simulink model "regulator_de_stare"  (R2023b)
settings: Solver=VariableStepAuto  StartTime=0.0  StopTime=200  RelTol=1e-3
settings Model: Creator=Iustin  LastModifiedBy=Iustin

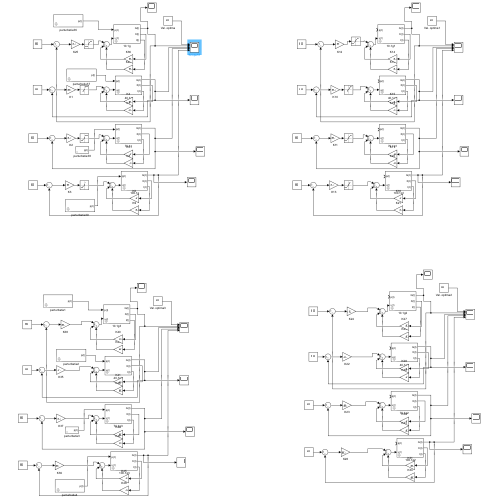
[thumbnail: Simulink's stored preview of the top-level diagram]
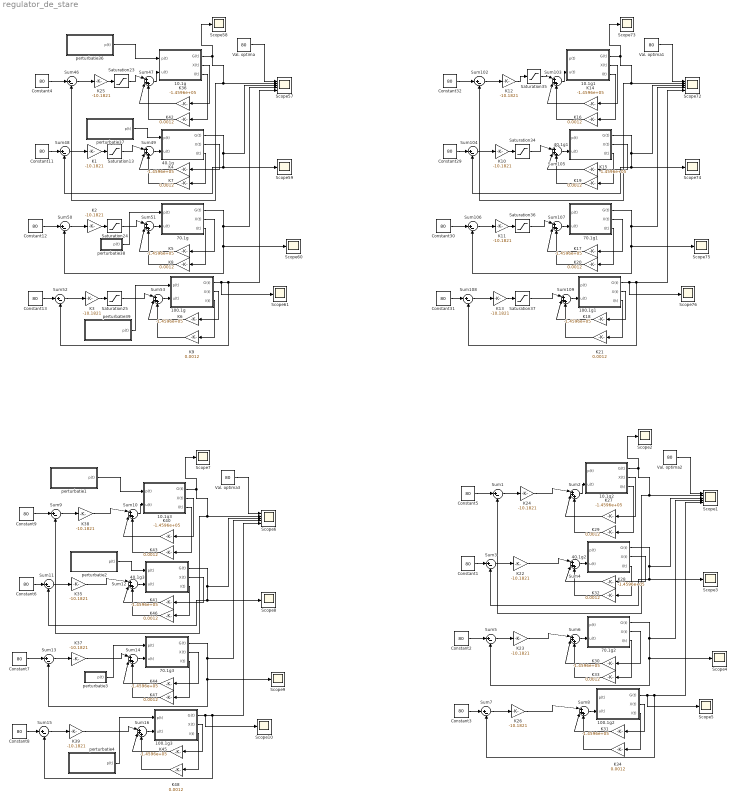
== system regulator_de_stare ==
  " 100.1g" : Subsystem  mask{Gb=80, V=120, p1=0.032, p2=0.019, p3=0.00000987, n=0.208, G0=100}
  " 100.1g1" : Subsystem  mask{Gb=80, V=120, p1=0.032, p2=0.019, p3=0.00000987, n=0.208, G0=300}
  " 100.1g2" : Subsystem  mask{Gb=80, V=120, p1=0.032, p2=0.019, p3=0.00000987, n=0.208, G0=300}
  " 100.1g3" : Subsystem  mask{Gb=80, V=120, p1=0.032, p2=0.019, p3=0.00000987, n=0.208, G0=100}
  10.1g : Subsystem  mask{Gb=80, V=120, p1=0.032, p2=0.019, p3=0.00000987, n=0.208, G0=100}
  10.1g1 : Subsystem  mask{Gb=80, V=120, p1=0.032, p2=0.019, p3=0.00000987, n=0.208, G0=150}
  10.1g2 : Subsystem  mask{Gb=80, V=120, p1=0.032, p2=0.019, p3=0.00000987, n=0.208, G0=150}
  10.1g3 : Subsystem  mask{Gb=80, V=120, p1=0.032, p2=0.019, p3=0.00000987, n=0.208, G0=100}
  40.1g : Subsystem  mask{Gb=80, V=120, p1=0.032, p2=0.019, p3=0.00000987, n=0.208, G0=100}
  40.1g1 : Subsystem  mask{Gb=80, V=120, p1=0.032, p2=0.019, p3=0.00000987, n=0.208, G0=200}
  40.1g2 : Subsystem  mask{Gb=80, V=120, p1=0.032, p2=0.019, p3=0.00000987, n=0.208, G0=200}
  40.1g3 : Subsystem  mask{Gb=80, V=120, p1=0.032, p2=0.019, p3=0.00000987, n=0.208, G0=100}
  70.1g : Subsystem  mask{Gb=80, V=120, p1=0.032, p2=0.019, p3=0.00000987, n=0.208, G0=100}
  70.1g1 : Subsystem  mask{Gb=80, V=120, p1=0.032, p2=0.019, p3=0.00000987, n=0.208, G0=250}
  70.1g2 : Subsystem  mask{Gb=80, V=120, p1=0.032, p2=0.019, p3=0.00000987, n=0.208, G0=250}
  70.1g3 : Subsystem  mask{Gb=80, V=120, p1=0.032, p2=0.019, p3=0.00000987, n=0.208, G0=100}
  Constant{1..9,11..13,29..32} (16 alike) : Constant  Value=80
  K{1..3,10..13,22..26,35,37..39} (16 alike) : Gain  Gain=-10.1821
  K{4..6,14..15,17..18,27..28,30..31,36,40..41,44..45} (16 alike) : Gain  Gain=-1.4596e+05
  K{7..9,16,19..21,29,32..34,42..43,46..48} (16 alike) : Gain  Gain=0.0012
  Saturation{13,23..25,34..37} (8 alike) : Saturate  UpperLimit=500  LowerLimit=0
  Scope{1,6,57,72} (4 alike) : Scope  NumInputPorts=5
  Scope{2..5,7..10,58..61,73..76} (16 alike) : Scope
  Sum{1,3,5,7,9,11,13,15,46,48,50,52,102,104,106,108} (16 alike) : Sum  Inputs=|+-
  Sum{2,4,6,8,10,12,14,16,47,49,51,53,103,105,107,109} (16 alike) : Sum  Inputs=|+++
  Val. optima{,1..3} (4 alike) : Constant  Value=80
  perturbatie1 : Subsystem  mask{Dg=10*1000, Ag=0.8, tg_max=40}
  perturbatie2 : Subsystem  mask{Dg=40*1000, Ag=0.8, tg_max=40}
  perturbatie3 : Subsystem  mask{Dg=70*1000, Ag=0.8, tg_max=40}
  perturbatie36 : Subsystem  mask{Dg=10*1000, Ag=0.8, tg_max=40}
  perturbatie37 : Subsystem  mask{Dg=40*1000, Ag=0.8, tg_max=40}
  perturbatie38 : Subsystem  mask{Dg=70*1000, Ag=0.8, tg_max=40}
  perturbatie39 : Subsystem  mask{Dg=100*1000, Ag=0.8, tg_max=40}
  perturbatie4 : Subsystem  mask{Dg=100*1000, Ag=0.8, tg_max=40}
  wires:
  70.1g1/2(X(t)) -> K17/1
  K16/1 -> Sum103/3
  40.1g1/2(X(t)) -> K15/1
  Sum107/1 -> 70.1g1/2(u(t))
  K19/1 -> Sum105/3
  K14/1 -> Sum103/2
  40.1g1/1(G(t)) -> Scope72/3, Scope74/1, Sum104/2
  Constant30/1 -> Sum106/1
  10.1g1/2(X(t)) -> K14/1
  Saturation34/1 -> Sum105/1
  " 100.1g1"/3(I(t)) -> K21/1
  70.1g1/1(G(t)) -> Scope72/4, Scope75/1, Sum106/2
  " 100.1g1"/2(X(t)) -> K18/1
  40.1g1/3(I(t)) -> K19/1
  Constant32/1 -> Sum102/1
  Sum103/1 -> 10.1g1/2(u(t))
  70.1g1/3(I(t)) -> K20/1
  " 100.1g1"/1(G(t)) -> Scope76/1, Scope72/5, Sum108/2
  Sum109/1 -> " 100.1g1"/2(u(t))
  Sum105/1 -> 40.1g1/2(u(t))
  Sum104/1 -> K10/1
  Constant31/1 -> Sum108/1
  K18/1 -> Sum109/2
  K10/1 -> Saturation34/1
  Sum106/1 -> K11/1
  10.1g1/1(G(t)) -> Sum102/2, Scope72/2, Scope73/1
  K11/1 -> Saturation36/1
  Val. optima1/1 -> Scope72/1
  Saturation37/1 -> Sum109/1
  K20/1 -> Sum107/3
  K8/1 -> Sum51/3
  K21/1 -> Sum109/3
  Sum108/1 -> K13/1
  Saturation36/1 -> Sum107/1
  K17/1 -> Sum107/2
  40.1g/3(I(t)) -> K7/1
  Sum51/1 -> 70.1g/2(u(t))
  10.1g/2(X(t)) -> K36/1
  70.1g/1(G(t)) -> Scope57/4, Scope60/1, Sum50/2
  Val. optima/1 -> Scope57/1
  Sum46/1 -> K25/1
  Saturation23/1 -> Sum47/1
  Saturation13/1 -> Sum49/1
  70.1g/3(I(t)) -> K8/1
  Constant4/1 -> Sum46/1
  Constant11/1 -> Sum48/1
  K4/1 -> Sum49/2
  70.1g/2(X(t)) -> K5/1
  K5/1 -> Sum51/2
  K15/1 -> Sum105/2
  Saturation25/1 -> Sum53/1
  K36/1 -> Sum47/2
  K3/1 -> Saturation25/1
  40.1g/1(G(t)) -> Scope57/3, Scope59/1, Sum48/2
  perturbatie39/1(p(t)) -> " 100.1g"/1(p(t))
  K6/1 -> Sum53/2
  Saturation24/1 -> Sum51/1
  K7/1 -> Sum49/3
  K25/1 -> Saturation23/1
  perturbatie38/1(p(t)) -> 70.1g/1(p(t))
  Sum102/1 -> K12/1
  perturbatie36/1(p(t)) -> 10.1g/1(p(t))
  K42/1 -> Sum47/3
  Constant12/1 -> Sum50/1
  10.1g/3(I(t)) -> K42/1
  Constant29/1 -> Sum104/1
  " 100.1g"/3(I(t)) -> K9/1
  Sum47/1 -> 10.1g/2(u(t))
  K9/1 -> Sum53/3
  K1/1 -> Saturation13/1
  Sum53/1 -> " 100.1g"/2(u(t))
  K2/1 -> Saturation24/1
  K13/1 -> Saturation37/1
  Sum49/1 -> 40.1g/2(u(t))
  Constant13/1 -> Sum52/1
  perturbatie37/1(p(t)) -> 40.1g/1(p(t))
  Sum52/1 -> K3/1
  40.1g/2(X(t)) -> K4/1
  " 100.1g"/2(X(t)) -> K6/1
  Sum48/1 -> K1/1
  Sum50/1 -> K2/1
  K12/1 -> Saturation35/1
  10.1g1/3(I(t)) -> K16/1
  10.1g/1(G(t)) -> Sum46/2, Scope57/2, Scope58/1
  Saturation35/1 -> Sum103/1
  " 100.1g"/1(G(t)) -> Scope61/1, Scope57/5, Sum52/2
  Sum4/1 -> 40.1g2/2(u(t))
  K23/1 -> Sum6/1
  K26/1 -> Sum8/1
  70.1g2/1(G(t)) -> Scope1/4, Scope4/1, Sum5/2
  Sum8/1 -> " 100.1g2"/2(u(t))
  " 100.1g2"/1(G(t)) -> Scope5/1, Scope1/5, Sum7/2
  70.1g2/3(I(t)) -> K33/1
  40.1g2/3(I(t)) -> K32/1
  Sum3/1 -> K22/1
  " 100.1g2"/3(I(t)) -> K34/1
  10.1g2/1(G(t)) -> Sum1/2, Scope1/2, Scope2/1
  Constant1/1 -> Sum3/1
  " 100.1g2"/2(X(t)) -> K31/1
  Sum5/1 -> K23/1
  Sum6/1 -> 70.1g2/2(u(t))
  K31/1 -> Sum8/2
  10.1g2/2(X(t)) -> K27/1
  40.1g2/1(G(t)) -> Scope1/3, Scope3/1, Sum3/2
  K28/1 -> Sum4/2
  K29/1 -> Sum2/3
  K22/1 -> Sum4/1
  K32/1 -> Sum4/3
  70.1g2/2(X(t)) -> K30/1
  40.1g2/2(X(t)) -> K28/1
  Constant5/1 -> Sum1/1
  Constant2/1 -> Sum5/1
  K27/1 -> Sum2/2
  K30/1 -> Sum6/2
  10.1g2/3(I(t)) -> K29/1
  Val. optima2/1 -> Scope1/1
  K33/1 -> Sum6/3
  K24/1 -> Sum2/1
  Sum1/1 -> K24/1
  Sum2/1 -> 10.1g2/2(u(t))
  Sum7/1 -> K26/1
  K34/1 -> Sum8/3
  Constant3/1 -> Sum7/1
  70.1g3/1(G(t)) -> Scope6/4, Scope9/1, Sum13/2
  Sum10/1 -> 10.1g3/2(u(t))
  " 100.1g3"/3(I(t)) -> K48/1
  Val. optima3/1 -> Scope6/1
  K35/1 -> Sum12/1
  40.1g3/3(I(t)) -> K46/1
  K38/1 -> Sum10/1
  Constant6/1 -> Sum11/1
  K39/1 -> Sum16/1
  K40/1 -> Sum10/2
  Sum13/1 -> K37/1
  K41/1 -> Sum12/2
  Sum11/1 -> K35/1
  Sum12/1 -> 40.1g3/2(u(t))
  Sum15/1 -> K39/1
  Sum16/1 -> " 100.1g3"/2(u(t))
  K46/1 -> Sum12/3
  40.1g3/1(G(t)) -> Scope6/3, Scope8/1, Sum11/2
  40.1g3/2(X(t)) -> K41/1
  Constant8/1 -> Sum15/1
  Sum9/1 -> K38/1
  perturbatie3/1(p(t)) -> 70.1g3/1(p(t))
  K44/1 -> Sum14/2
  70.1g3/3(I(t)) -> K47/1
  Constant7/1 -> Sum13/1
  K37/1 -> Sum14/1
  K43/1 -> Sum10/3
  perturbatie4/1(p(t)) -> " 100.1g3"/1(p(t))
  10.1g3/2(X(t)) -> K40/1
  K47/1 -> Sum14/3
  Constant9/1 -> Sum9/1
  " 100.1g3"/2(X(t)) -> K45/1
  10.1g3/1(G(t)) -> Sum9/2, Scope6/2, Scope7/1
  K45/1 -> Sum16/2
  perturbatie2/1(p(t)) -> 40.1g3/1(p(t))
  Sum14/1 -> 70.1g3/2(u(t))
  10.1g3/3(I(t)) -> K43/1
  perturbatie1/1(p(t)) -> 10.1g3/1(p(t))
  " 100.1g3"/1(G(t)) -> Scope10/1, Scope6/5, Sum15/2
  70.1g3/2(X(t)) -> K44/1
  K48/1 -> Sum16/3

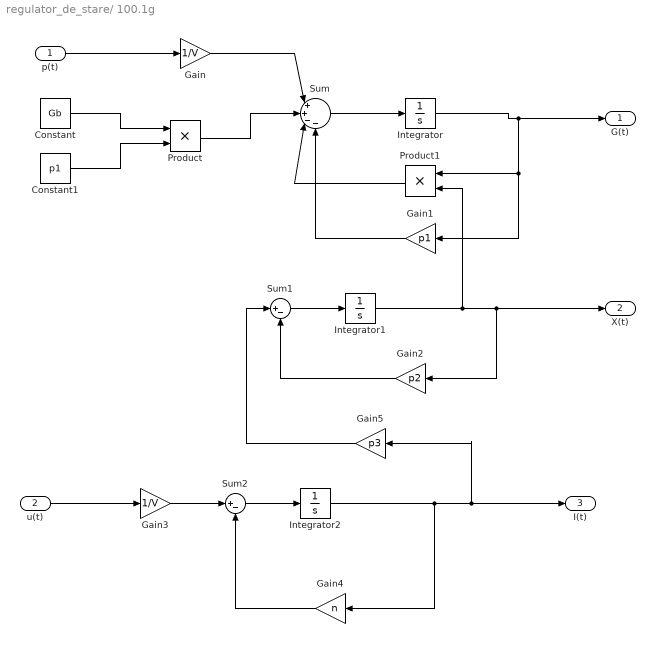
== system regulator_de_stare/ 100.1g ==
  p(t) : Inport
  u(t) : Inport  Port=2
  Constant : Constant  Value=Gb
  Constant1 : Constant  Value=p1
  Gain : Gain  Gain=1/V
  Gain1 : Gain  Gain=p1
  Gain2 : Gain  Gain=p2
  Gain3 : Gain  Gain=1/V
  Gain4 : Gain  Gain=n
  Gain5 : Gain  Gain=p3
  Integrator : Integrator  InitialCondition=G0
  Integrator1 : Integrator
  Integrator2 : Integrator
  Product : Product
  Product1 : Product
  Sum : Sum  Inputs=|++--
  Sum1 : Sum  Inputs=|+-
  Sum2 : Sum  Inputs=|+-
  G(t) : Outport
  X(t) : Outport  Port=2
  I(t) : Outport  Port=3
  wires:
  Sum2/1 -> Integrator2/1
  Gain3/1 -> Sum2/1
  Sum1/1 -> Integrator1/1
  Integrator2/1 -> Gain4/1, I(t)/1, Gain5/1
  u(t)/1 -> Gain3/1
  Integrator1/1 -> Product1/2, X(t)/1, Gain2/1
  Product/1 -> Sum/2
  Integrator/1 -> G(t)/1, Gain1/1, Product1/1
  Gain5/1 -> Sum1/1
  Sum/1 -> Integrator/1
  Constant1/1 -> Product/2
  Constant/1 -> Product/1
  Gain4/1 -> Sum2/2
  Gain2/1 -> Sum1/2
  Product1/1 -> Sum/3
  Gain1/1 -> Sum/4
  p(t)/1 -> Gain/1
  Gain/1 -> Sum/1

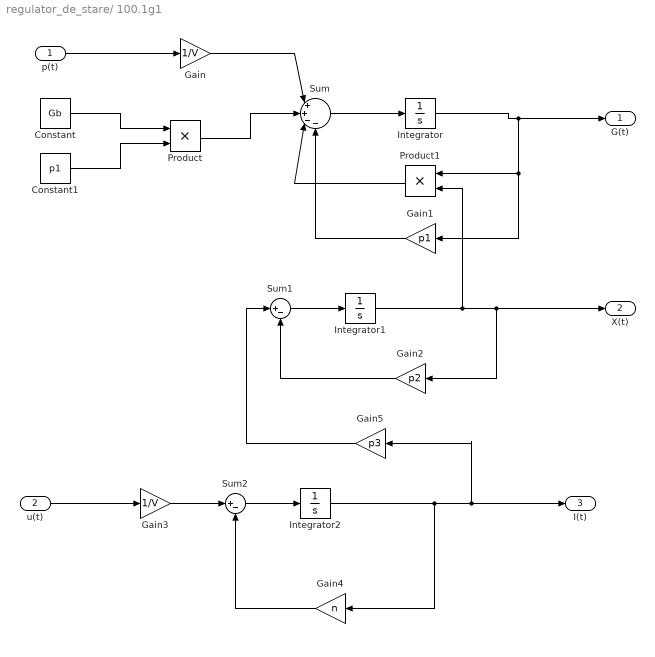
== system regulator_de_stare/ 100.1g1 ==
  p(t) : Inport
  u(t) : Inport  Port=2
  Constant : Constant  Value=Gb
  Constant1 : Constant  Value=p1
  Gain : Gain  Gain=1/V
  Gain1 : Gain  Gain=p1
  Gain2 : Gain  Gain=p2
  Gain3 : Gain  Gain=1/V
  Gain4 : Gain  Gain=n
  Gain5 : Gain  Gain=p3
  Integrator : Integrator  InitialCondition=G0
  Integrator1 : Integrator
  Integrator2 : Integrator
  Product : Product
  Product1 : Product
  Sum : Sum  Inputs=|++--
  Sum1 : Sum  Inputs=|+-
  Sum2 : Sum  Inputs=|+-
  G(t) : Outport
  X(t) : Outport  Port=2
  I(t) : Outport  Port=3
  wires:
  Sum2/1 -> Integrator2/1
  Gain3/1 -> Sum2/1
  Sum1/1 -> Integrator1/1
  Integrator2/1 -> Gain4/1, I(t)/1, Gain5/1
  u(t)/1 -> Gain3/1
  Integrator1/1 -> Product1/2, X(t)/1, Gain2/1
  Product/1 -> Sum/2
  Integrator/1 -> G(t)/1, Gain1/1, Product1/1
  Gain5/1 -> Sum1/1
  Sum/1 -> Integrator/1
  Constant1/1 -> Product/2
  Constant/1 -> Product/1
  Gain4/1 -> Sum2/2
  Gain2/1 -> Sum1/2
  Product1/1 -> Sum/3
  Gain1/1 -> Sum/4
  p(t)/1 -> Gain/1
  Gain/1 -> Sum/1

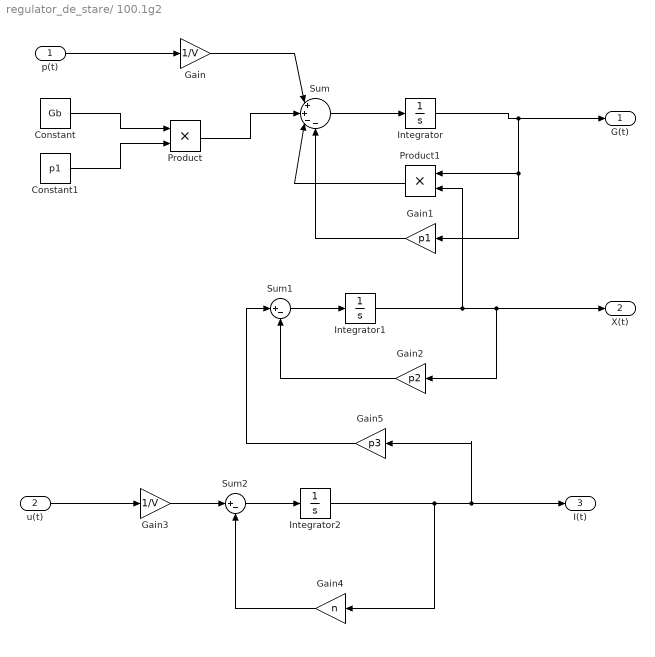
== system regulator_de_stare/ 100.1g2 ==
  p(t) : Inport
  u(t) : Inport  Port=2
  Constant : Constant  Value=Gb
  Constant1 : Constant  Value=p1
  Gain : Gain  Gain=1/V
  Gain1 : Gain  Gain=p1
  Gain2 : Gain  Gain=p2
  Gain3 : Gain  Gain=1/V
  Gain4 : Gain  Gain=n
  Gain5 : Gain  Gain=p3
  Integrator : Integrator  InitialCondition=G0
  Integrator1 : Integrator
  Integrator2 : Integrator
  Product : Product
  Product1 : Product
  Sum : Sum  Inputs=|++--
  Sum1 : Sum  Inputs=|+-
  Sum2 : Sum  Inputs=|+-
  G(t) : Outport
  X(t) : Outport  Port=2
  I(t) : Outport  Port=3
  wires:
  Sum2/1 -> Integrator2/1
  Gain3/1 -> Sum2/1
  Sum1/1 -> Integrator1/1
  Integrator2/1 -> Gain4/1, I(t)/1, Gain5/1
  u(t)/1 -> Gain3/1
  Integrator1/1 -> Product1/2, X(t)/1, Gain2/1
  Product/1 -> Sum/2
  Integrator/1 -> G(t)/1, Gain1/1, Product1/1
  Gain5/1 -> Sum1/1
  Sum/1 -> Integrator/1
  Constant1/1 -> Product/2
  Constant/1 -> Product/1
  Gain4/1 -> Sum2/2
  Gain2/1 -> Sum1/2
  Product1/1 -> Sum/3
  Gain1/1 -> Sum/4
  p(t)/1 -> Gain/1
  Gain/1 -> Sum/1

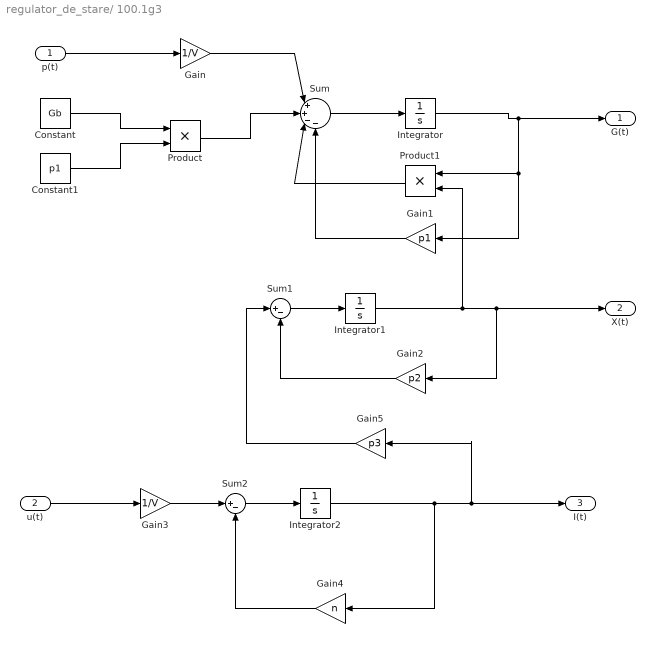
== system regulator_de_stare/ 100.1g3 ==
  p(t) : Inport
  u(t) : Inport  Port=2
  Constant : Constant  Value=Gb
  Constant1 : Constant  Value=p1
  Gain : Gain  Gain=1/V
  Gain1 : Gain  Gain=p1
  Gain2 : Gain  Gain=p2
  Gain3 : Gain  Gain=1/V
  Gain4 : Gain  Gain=n
  Gain5 : Gain  Gain=p3
  Integrator : Integrator  InitialCondition=G0
  Integrator1 : Integrator
  Integrator2 : Integrator
  Product : Product
  Product1 : Product
  Sum : Sum  Inputs=|++--
  Sum1 : Sum  Inputs=|+-
  Sum2 : Sum  Inputs=|+-
  G(t) : Outport
  X(t) : Outport  Port=2
  I(t) : Outport  Port=3
  wires:
  Sum2/1 -> Integrator2/1
  Gain3/1 -> Sum2/1
  Sum1/1 -> Integrator1/1
  Integrator2/1 -> Gain4/1, I(t)/1, Gain5/1
  u(t)/1 -> Gain3/1
  Integrator1/1 -> Product1/2, X(t)/1, Gain2/1
  Product/1 -> Sum/2
  Integrator/1 -> G(t)/1, Gain1/1, Product1/1
  Gain5/1 -> Sum1/1
  Sum/1 -> Integrator/1
  Constant1/1 -> Product/2
  Constant/1 -> Product/1
  Gain4/1 -> Sum2/2
  Gain2/1 -> Sum1/2
  Product1/1 -> Sum/3
  Gain1/1 -> Sum/4
  p(t)/1 -> Gain/1
  Gain/1 -> Sum/1

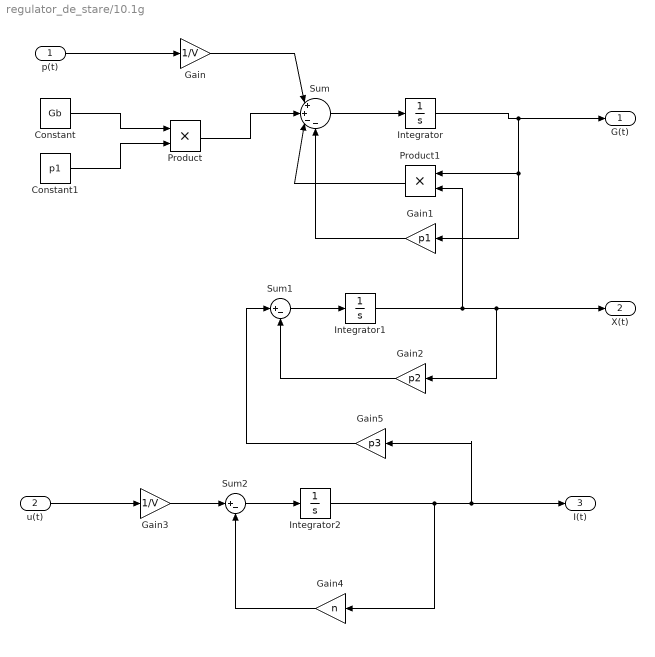
== system regulator_de_stare/10.1g ==
  p(t) : Inport
  u(t) : Inport  Port=2
  Constant : Constant  Value=Gb
  Constant1 : Constant  Value=p1
  Gain : Gain  Gain=1/V
  Gain1 : Gain  Gain=p1
  Gain2 : Gain  Gain=p2
  Gain3 : Gain  Gain=1/V
  Gain4 : Gain  Gain=n
  Gain5 : Gain  Gain=p3
  Integrator : Integrator  InitialCondition=G0
  Integrator1 : Integrator
  Integrator2 : Integrator
  Product : Product
  Product1 : Product
  Sum : Sum  Inputs=|++--
  Sum1 : Sum  Inputs=|+-
  Sum2 : Sum  Inputs=|+-
  G(t) : Outport
  X(t) : Outport  Port=2
  I(t) : Outport  Port=3
  wires:
  Sum2/1 -> Integrator2/1
  Gain3/1 -> Sum2/1
  Sum1/1 -> Integrator1/1
  Integrator2/1 -> Gain4/1, I(t)/1, Gain5/1
  u(t)/1 -> Gain3/1
  Integrator1/1 -> Product1/2, X(t)/1, Gain2/1
  Product/1 -> Sum/2
  Integrator/1 -> G(t)/1, Gain1/1, Product1/1
  Gain5/1 -> Sum1/1
  Sum/1 -> Integrator/1
  Constant1/1 -> Product/2
  Constant/1 -> Product/1
  Gain4/1 -> Sum2/2
  Gain2/1 -> Sum1/2
  Product1/1 -> Sum/3
  Gain1/1 -> Sum/4
  p(t)/1 -> Gain/1
  Gain/1 -> Sum/1

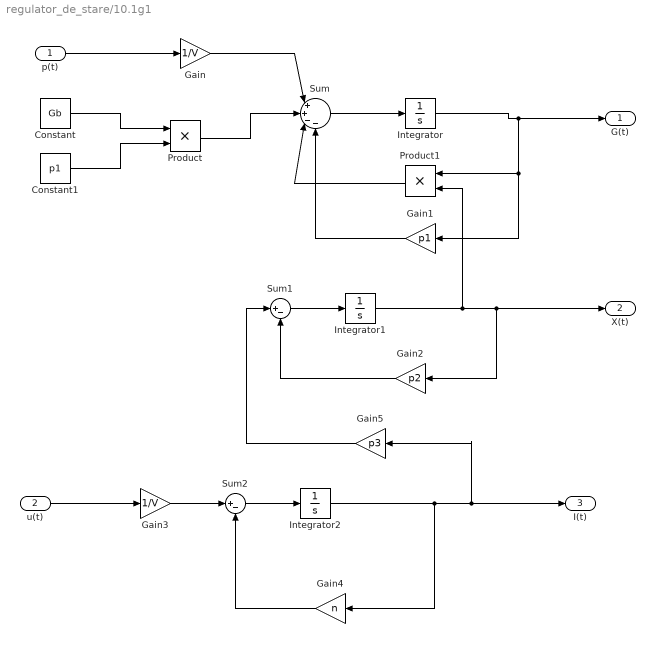
== system regulator_de_stare/10.1g1 ==
  p(t) : Inport
  u(t) : Inport  Port=2
  Constant : Constant  Value=Gb
  Constant1 : Constant  Value=p1
  Gain : Gain  Gain=1/V
  Gain1 : Gain  Gain=p1
  Gain2 : Gain  Gain=p2
  Gain3 : Gain  Gain=1/V
  Gain4 : Gain  Gain=n
  Gain5 : Gain  Gain=p3
  Integrator : Integrator  InitialCondition=G0
  Integrator1 : Integrator
  Integrator2 : Integrator
  Product : Product
  Product1 : Product
  Sum : Sum  Inputs=|++--
  Sum1 : Sum  Inputs=|+-
  Sum2 : Sum  Inputs=|+-
  G(t) : Outport
  X(t) : Outport  Port=2
  I(t) : Outport  Port=3
  wires:
  Sum2/1 -> Integrator2/1
  Gain3/1 -> Sum2/1
  Sum1/1 -> Integrator1/1
  Integrator2/1 -> Gain4/1, I(t)/1, Gain5/1
  u(t)/1 -> Gain3/1
  Integrator1/1 -> Product1/2, X(t)/1, Gain2/1
  Product/1 -> Sum/2
  Integrator/1 -> G(t)/1, Gain1/1, Product1/1
  Gain5/1 -> Sum1/1
  Sum/1 -> Integrator/1
  Constant1/1 -> Product/2
  Constant/1 -> Product/1
  Gain4/1 -> Sum2/2
  Gain2/1 -> Sum1/2
  Product1/1 -> Sum/3
  Gain1/1 -> Sum/4
  p(t)/1 -> Gain/1
  Gain/1 -> Sum/1

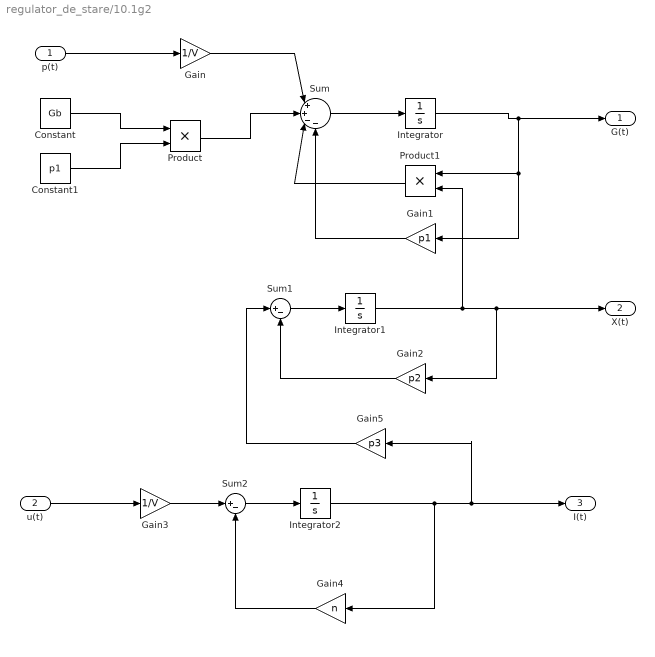
== system regulator_de_stare/10.1g2 ==
  p(t) : Inport
  u(t) : Inport  Port=2
  Constant : Constant  Value=Gb
  Constant1 : Constant  Value=p1
  Gain : Gain  Gain=1/V
  Gain1 : Gain  Gain=p1
  Gain2 : Gain  Gain=p2
  Gain3 : Gain  Gain=1/V
  Gain4 : Gain  Gain=n
  Gain5 : Gain  Gain=p3
  Integrator : Integrator  InitialCondition=G0
  Integrator1 : Integrator
  Integrator2 : Integrator
  Product : Product
  Product1 : Product
  Sum : Sum  Inputs=|++--
  Sum1 : Sum  Inputs=|+-
  Sum2 : Sum  Inputs=|+-
  G(t) : Outport
  X(t) : Outport  Port=2
  I(t) : Outport  Port=3
  wires:
  Sum2/1 -> Integrator2/1
  Gain3/1 -> Sum2/1
  Sum1/1 -> Integrator1/1
  Integrator2/1 -> Gain4/1, I(t)/1, Gain5/1
  u(t)/1 -> Gain3/1
  Integrator1/1 -> Product1/2, X(t)/1, Gain2/1
  Product/1 -> Sum/2
  Integrator/1 -> G(t)/1, Gain1/1, Product1/1
  Gain5/1 -> Sum1/1
  Sum/1 -> Integrator/1
  Constant1/1 -> Product/2
  Constant/1 -> Product/1
  Gain4/1 -> Sum2/2
  Gain2/1 -> Sum1/2
  Product1/1 -> Sum/3
  Gain1/1 -> Sum/4
  p(t)/1 -> Gain/1
  Gain/1 -> Sum/1

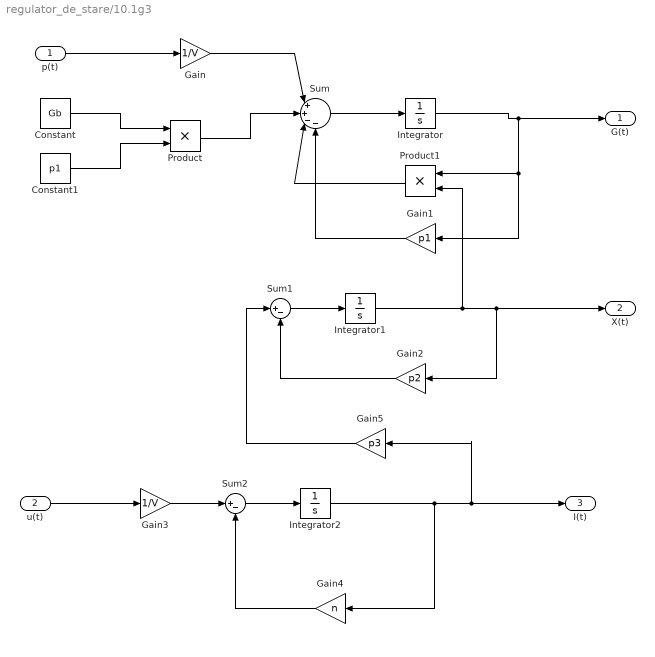
== system regulator_de_stare/10.1g3 ==
  p(t) : Inport
  u(t) : Inport  Port=2
  Constant : Constant  Value=Gb
  Constant1 : Constant  Value=p1
  Gain : Gain  Gain=1/V
  Gain1 : Gain  Gain=p1
  Gain2 : Gain  Gain=p2
  Gain3 : Gain  Gain=1/V
  Gain4 : Gain  Gain=n
  Gain5 : Gain  Gain=p3
  Integrator : Integrator  InitialCondition=G0
  Integrator1 : Integrator
  Integrator2 : Integrator
  Product : Product
  Product1 : Product
  Sum : Sum  Inputs=|++--
  Sum1 : Sum  Inputs=|+-
  Sum2 : Sum  Inputs=|+-
  G(t) : Outport
  X(t) : Outport  Port=2
  I(t) : Outport  Port=3
  wires:
  Sum2/1 -> Integrator2/1
  Gain3/1 -> Sum2/1
  Sum1/1 -> Integrator1/1
  Integrator2/1 -> Gain4/1, I(t)/1, Gain5/1
  u(t)/1 -> Gain3/1
  Integrator1/1 -> Product1/2, X(t)/1, Gain2/1
  Product/1 -> Sum/2
  Integrator/1 -> G(t)/1, Gain1/1, Product1/1
  Gain5/1 -> Sum1/1
  Sum/1 -> Integrator/1
  Constant1/1 -> Product/2
  Constant/1 -> Product/1
  Gain4/1 -> Sum2/2
  Gain2/1 -> Sum1/2
  Product1/1 -> Sum/3
  Gain1/1 -> Sum/4
  p(t)/1 -> Gain/1
  Gain/1 -> Sum/1

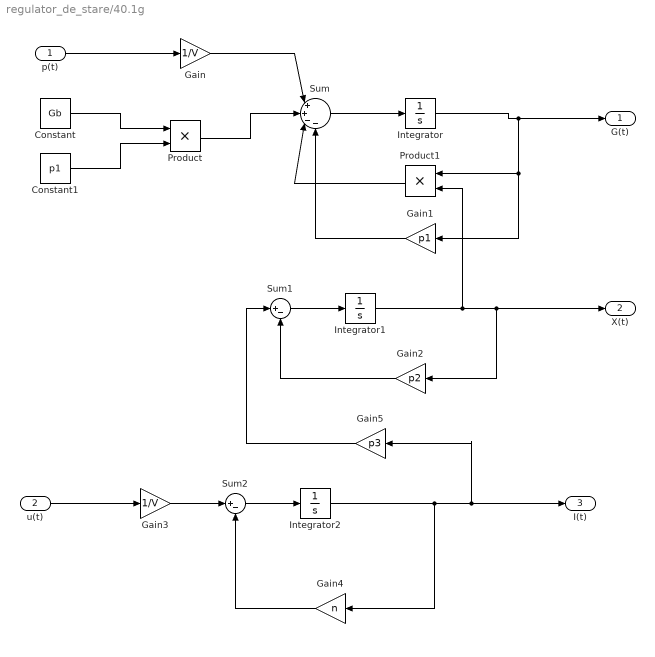
== system regulator_de_stare/40.1g ==
  p(t) : Inport
  u(t) : Inport  Port=2
  Constant : Constant  Value=Gb
  Constant1 : Constant  Value=p1
  Gain : Gain  Gain=1/V
  Gain1 : Gain  Gain=p1
  Gain2 : Gain  Gain=p2
  Gain3 : Gain  Gain=1/V
  Gain4 : Gain  Gain=n
  Gain5 : Gain  Gain=p3
  Integrator : Integrator  InitialCondition=G0
  Integrator1 : Integrator
  Integrator2 : Integrator
  Product : Product
  Product1 : Product
  Sum : Sum  Inputs=|++--
  Sum1 : Sum  Inputs=|+-
  Sum2 : Sum  Inputs=|+-
  G(t) : Outport
  X(t) : Outport  Port=2
  I(t) : Outport  Port=3
  wires:
  Sum2/1 -> Integrator2/1
  Gain3/1 -> Sum2/1
  Sum1/1 -> Integrator1/1
  Integrator2/1 -> Gain4/1, I(t)/1, Gain5/1
  u(t)/1 -> Gain3/1
  Integrator1/1 -> Product1/2, X(t)/1, Gain2/1
  Product/1 -> Sum/2
  Integrator/1 -> G(t)/1, Gain1/1, Product1/1
  Gain5/1 -> Sum1/1
  Sum/1 -> Integrator/1
  Constant1/1 -> Product/2
  Constant/1 -> Product/1
  Gain4/1 -> Sum2/2
  Gain2/1 -> Sum1/2
  Product1/1 -> Sum/3
  Gain1/1 -> Sum/4
  p(t)/1 -> Gain/1
  Gain/1 -> Sum/1

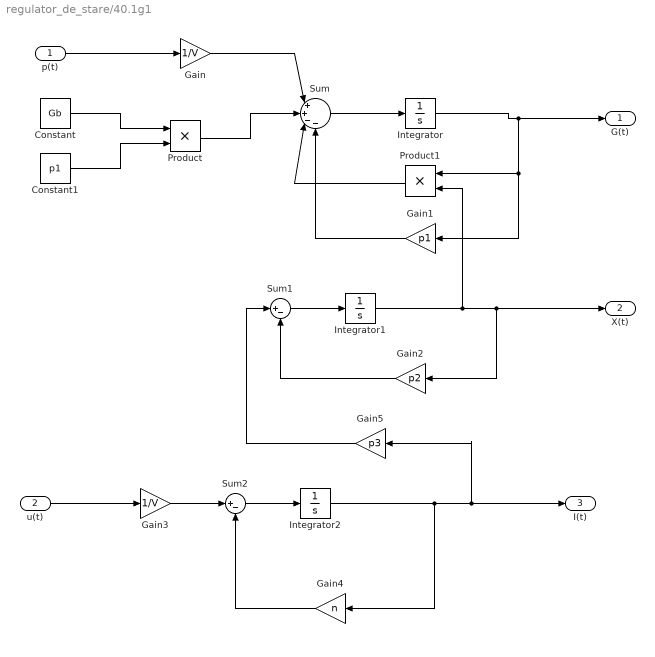
== system regulator_de_stare/40.1g1 ==
  p(t) : Inport
  u(t) : Inport  Port=2
  Constant : Constant  Value=Gb
  Constant1 : Constant  Value=p1
  Gain : Gain  Gain=1/V
  Gain1 : Gain  Gain=p1
  Gain2 : Gain  Gain=p2
  Gain3 : Gain  Gain=1/V
  Gain4 : Gain  Gain=n
  Gain5 : Gain  Gain=p3
  Integrator : Integrator  InitialCondition=G0
  Integrator1 : Integrator
  Integrator2 : Integrator
  Product : Product
  Product1 : Product
  Sum : Sum  Inputs=|++--
  Sum1 : Sum  Inputs=|+-
  Sum2 : Sum  Inputs=|+-
  G(t) : Outport
  X(t) : Outport  Port=2
  I(t) : Outport  Port=3
  wires:
  Sum2/1 -> Integrator2/1
  Gain3/1 -> Sum2/1
  Sum1/1 -> Integrator1/1
  Integrator2/1 -> Gain4/1, I(t)/1, Gain5/1
  u(t)/1 -> Gain3/1
  Integrator1/1 -> Product1/2, X(t)/1, Gain2/1
  Product/1 -> Sum/2
  Integrator/1 -> G(t)/1, Gain1/1, Product1/1
  Gain5/1 -> Sum1/1
  Sum/1 -> Integrator/1
  Constant1/1 -> Product/2
  Constant/1 -> Product/1
  Gain4/1 -> Sum2/2
  Gain2/1 -> Sum1/2
  Product1/1 -> Sum/3
  Gain1/1 -> Sum/4
  p(t)/1 -> Gain/1
  Gain/1 -> Sum/1

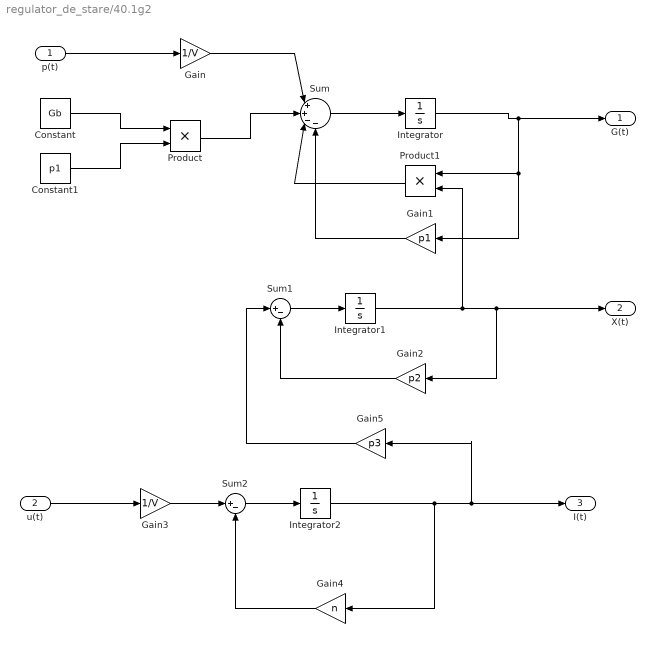
== system regulator_de_stare/40.1g2 ==
  p(t) : Inport
  u(t) : Inport  Port=2
  Constant : Constant  Value=Gb
  Constant1 : Constant  Value=p1
  Gain : Gain  Gain=1/V
  Gain1 : Gain  Gain=p1
  Gain2 : Gain  Gain=p2
  Gain3 : Gain  Gain=1/V
  Gain4 : Gain  Gain=n
  Gain5 : Gain  Gain=p3
  Integrator : Integrator  InitialCondition=G0
  Integrator1 : Integrator
  Integrator2 : Integrator
  Product : Product
  Product1 : Product
  Sum : Sum  Inputs=|++--
  Sum1 : Sum  Inputs=|+-
  Sum2 : Sum  Inputs=|+-
  G(t) : Outport
  X(t) : Outport  Port=2
  I(t) : Outport  Port=3
  wires:
  Sum2/1 -> Integrator2/1
  Gain3/1 -> Sum2/1
  Sum1/1 -> Integrator1/1
  Integrator2/1 -> Gain4/1, I(t)/1, Gain5/1
  u(t)/1 -> Gain3/1
  Integrator1/1 -> Product1/2, X(t)/1, Gain2/1
  Product/1 -> Sum/2
  Integrator/1 -> G(t)/1, Gain1/1, Product1/1
  Gain5/1 -> Sum1/1
  Sum/1 -> Integrator/1
  Constant1/1 -> Product/2
  Constant/1 -> Product/1
  Gain4/1 -> Sum2/2
  Gain2/1 -> Sum1/2
  Product1/1 -> Sum/3
  Gain1/1 -> Sum/4
  p(t)/1 -> Gain/1
  Gain/1 -> Sum/1

== system regulator_de_stare/40.1g3 ==
  p(t) : Inport
  u(t) : Inport  Port=2
  Constant : Constant  Value=Gb
  Constant1 : Constant  Value=p1
  Gain : Gain  Gain=1/V
  Gain1 : Gain  Gain=p1
  Gain2 : Gain  Gain=p2
  Gain3 : Gain  Gain=1/V
  Gain4 : Gain  Gain=n
  Gain5 : Gain  Gain=p3
  Integrator : Integrator  InitialCondition=G0
  Integrator1 : Integrator
  Integrator2 : Integrator
  Product : Product
  Product1 : Product
  Sum : Sum  Inputs=|++--
  Sum1 : Sum  Inputs=|+-
  Sum2 : Sum  Inputs=|+-
  G(t) : Outport
  X(t) : Outport  Port=2
  I(t) : Outport  Port=3
  wires:
  Sum2/1 -> Integrator2/1
  Gain3/1 -> Sum2/1
  Sum1/1 -> Integrator1/1
  Integrator2/1 -> Gain4/1, I(t)/1, Gain5/1
  u(t)/1 -> Gain3/1
  Integrator1/1 -> Product1/2, X(t)/1, Gain2/1
  Product/1 -> Sum/2
  Integrator/1 -> G(t)/1, Gain1/1, Product1/1
  Gain5/1 -> Sum1/1
  Sum/1 -> Integrator/1
  Constant1/1 -> Product/2
  Constant/1 -> Product/1
  Gain4/1 -> Sum2/2
  Gain2/1 -> Sum1/2
  Product1/1 -> Sum/3
  Gain1/1 -> Sum/4
  p(t)/1 -> Gain/1
  Gain/1 -> Sum/1

== system regulator_de_stare/70.1g ==
  p(t) : Inport
  u(t) : Inport  Port=2
  Constant : Constant  Value=Gb
  Constant1 : Constant  Value=p1
  Gain : Gain  Gain=1/V
  Gain1 : Gain  Gain=p1
  Gain2 : Gain  Gain=p2
  Gain3 : Gain  Gain=1/V
  Gain4 : Gain  Gain=n
  Gain5 : Gain  Gain=p3
  Integrator : Integrator  InitialCondition=G0
  Integrator1 : Integrator
  Integrator2 : Integrator
  Product : Product
  Product1 : Product
  Sum : Sum  Inputs=|++--
  Sum1 : Sum  Inputs=|+-
  Sum2 : Sum  Inputs=|+-
  G(t) : Outport
  X(t) : Outport  Port=2
  I(t) : Outport  Port=3
  wires:
  Sum2/1 -> Integrator2/1
  Gain3/1 -> Sum2/1
  Sum1/1 -> Integrator1/1
  Integrator2/1 -> Gain4/1, I(t)/1, Gain5/1
  u(t)/1 -> Gain3/1
  Integrator1/1 -> Product1/2, X(t)/1, Gain2/1
  Product/1 -> Sum/2
  Integrator/1 -> G(t)/1, Gain1/1, Product1/1
  Gain5/1 -> Sum1/1
  Sum/1 -> Integrator/1
  Constant1/1 -> Product/2
  Constant/1 -> Product/1
  Gain4/1 -> Sum2/2
  Gain2/1 -> Sum1/2
  Product1/1 -> Sum/3
  Gain1/1 -> Sum/4
  p(t)/1 -> Gain/1
  Gain/1 -> Sum/1

== system regulator_de_stare/70.1g1 ==
  p(t) : Inport
  u(t) : Inport  Port=2
  Constant : Constant  Value=Gb
  Constant1 : Constant  Value=p1
  Gain : Gain  Gain=1/V
  Gain1 : Gain  Gain=p1
  Gain2 : Gain  Gain=p2
  Gain3 : Gain  Gain=1/V
  Gain4 : Gain  Gain=n
  Gain5 : Gain  Gain=p3
  Integrator : Integrator  InitialCondition=G0
  Integrator1 : Integrator
  Integrator2 : Integrator
  Product : Product
  Product1 : Product
  Sum : Sum  Inputs=|++--
  Sum1 : Sum  Inputs=|+-
  Sum2 : Sum  Inputs=|+-
  G(t) : Outport
  X(t) : Outport  Port=2
  I(t) : Outport  Port=3
  wires:
  Sum2/1 -> Integrator2/1
  Gain3/1 -> Sum2/1
  Sum1/1 -> Integrator1/1
  Integrator2/1 -> Gain4/1, I(t)/1, Gain5/1
  u(t)/1 -> Gain3/1
  Integrator1/1 -> Product1/2, X(t)/1, Gain2/1
  Product/1 -> Sum/2
  Integrator/1 -> G(t)/1, Gain1/1, Product1/1
  Gain5/1 -> Sum1/1
  Sum/1 -> Integrator/1
  Constant1/1 -> Product/2
  Constant/1 -> Product/1
  Gain4/1 -> Sum2/2
  Gain2/1 -> Sum1/2
  Product1/1 -> Sum/3
  Gain1/1 -> Sum/4
  p(t)/1 -> Gain/1
  Gain/1 -> Sum/1

== system regulator_de_stare/70.1g2 ==
  p(t) : Inport
  u(t) : Inport  Port=2
  Constant : Constant  Value=Gb
  Constant1 : Constant  Value=p1
  Gain : Gain  Gain=1/V
  Gain1 : Gain  Gain=p1
  Gain2 : Gain  Gain=p2
  Gain3 : Gain  Gain=1/V
  Gain4 : Gain  Gain=n
  Gain5 : Gain  Gain=p3
  Integrator : Integrator  InitialCondition=G0
  Integrator1 : Integrator
  Integrator2 : Integrator
  Product : Product
  Product1 : Product
  Sum : Sum  Inputs=|++--
  Sum1 : Sum  Inputs=|+-
  Sum2 : Sum  Inputs=|+-
  G(t) : Outport
  X(t) : Outport  Port=2
  I(t) : Outport  Port=3
  wires:
  Sum2/1 -> Integrator2/1
  Gain3/1 -> Sum2/1
  Sum1/1 -> Integrator1/1
  Integrator2/1 -> Gain4/1, I(t)/1, Gain5/1
  u(t)/1 -> Gain3/1
  Integrator1/1 -> Product1/2, X(t)/1, Gain2/1
  Product/1 -> Sum/2
  Integrator/1 -> G(t)/1, Gain1/1, Product1/1
  Gain5/1 -> Sum1/1
  Sum/1 -> Integrator/1
  Constant1/1 -> Product/2
  Constant/1 -> Product/1
  Gain4/1 -> Sum2/2
  Gain2/1 -> Sum1/2
  Product1/1 -> Sum/3
  Gain1/1 -> Sum/4
  p(t)/1 -> Gain/1
  Gain/1 -> Sum/1

== system regulator_de_stare/70.1g3 ==
  p(t) : Inport
  u(t) : Inport  Port=2
  Constant : Constant  Value=Gb
  Constant1 : Constant  Value=p1
  Gain : Gain  Gain=1/V
  Gain1 : Gain  Gain=p1
  Gain2 : Gain  Gain=p2
  Gain3 : Gain  Gain=1/V
  Gain4 : Gain  Gain=n
  Gain5 : Gain  Gain=p3
  Integrator : Integrator  InitialCondition=G0
  Integrator1 : Integrator
  Integrator2 : Integrator
  Product : Product
  Product1 : Product
  Sum : Sum  Inputs=|++--
  Sum1 : Sum  Inputs=|+-
  Sum2 : Sum  Inputs=|+-
  G(t) : Outport
  X(t) : Outport  Port=2
  I(t) : Outport  Port=3
  wires:
  Sum2/1 -> Integrator2/1
  Gain3/1 -> Sum2/1
  Sum1/1 -> Integrator1/1
  Integrator2/1 -> Gain4/1, I(t)/1, Gain5/1
  u(t)/1 -> Gain3/1
  Integrator1/1 -> Product1/2, X(t)/1, Gain2/1
  Product/1 -> Sum/2
  Integrator/1 -> G(t)/1, Gain1/1, Product1/1
  Gain5/1 -> Sum1/1
  Sum/1 -> Integrator/1
  Constant1/1 -> Product/2
  Constant/1 -> Product/1
  Gain4/1 -> Sum2/2
  Gain2/1 -> Sum1/2
  Product1/1 -> Sum/3
  Gain1/1 -> Sum/4
  p(t)/1 -> Gain/1
  Gain/1 -> Sum/1

== system regulator_de_stare/perturbatie1 ==
  Clock : Clock
  Constant : Constant  Value=Dg
  Constant1 : Constant  Value=Ag
  Gain : Gain  Gain=-1/tg_max
  Gain1 : Gain  Gain=1/(tg_max*tg_max)
  Math Function : Math
  Product : Product  Inputs=4
  p(t) : Outport
  wires:
  Constant/1 -> Product/1
  Constant1/1 -> Product/2
  Clock/1 -> Gain/1, Product/3
  Gain/1 -> Math Function/1
  Math Function/1 -> Product/4
  Product/1 -> Gain1/1
  Gain1/1 -> p(t)/1

== system regulator_de_stare/perturbatie2 ==
  Clock : Clock
  Constant : Constant  Value=Dg
  Constant1 : Constant  Value=Ag
  Gain : Gain  Gain=-1/tg_max
  Gain1 : Gain  Gain=1/(tg_max*tg_max)
  Math Function : Math
  Product : Product  Inputs=4
  p(t) : Outport
  wires:
  Constant/1 -> Product/1
  Constant1/1 -> Product/2
  Clock/1 -> Gain/1, Product/3
  Gain/1 -> Math Function/1
  Math Function/1 -> Product/4
  Product/1 -> Gain1/1
  Gain1/1 -> p(t)/1

== system regulator_de_stare/perturbatie3 ==
  Clock : Clock
  Constant : Constant  Value=Dg
  Constant1 : Constant  Value=Ag
  Gain : Gain  Gain=-1/tg_max
  Gain1 : Gain  Gain=1/(tg_max*tg_max)
  Math Function : Math
  Product : Product  Inputs=4
  p(t) : Outport
  wires:
  Constant/1 -> Product/1
  Constant1/1 -> Product/2
  Clock/1 -> Gain/1, Product/3
  Gain/1 -> Math Function/1
  Math Function/1 -> Product/4
  Product/1 -> Gain1/1
  Gain1/1 -> p(t)/1

== system regulator_de_stare/perturbatie36 ==
  Clock : Clock
  Constant : Constant  Value=Dg
  Constant1 : Constant  Value=Ag
  Gain : Gain  Gain=-1/tg_max
  Gain1 : Gain  Gain=1/(tg_max*tg_max)
  Math Function : Math
  Product : Product  Inputs=4
  p(t) : Outport
  wires:
  Constant/1 -> Product/1
  Constant1/1 -> Product/2
  Clock/1 -> Gain/1, Product/3
  Gain/1 -> Math Function/1
  Math Function/1 -> Product/4
  Product/1 -> Gain1/1
  Gain1/1 -> p(t)/1

== system regulator_de_stare/perturbatie37 ==
  Clock : Clock
  Constant : Constant  Value=Dg
  Constant1 : Constant  Value=Ag
  Gain : Gain  Gain=-1/tg_max
  Gain1 : Gain  Gain=1/(tg_max*tg_max)
  Math Function : Math
  Product : Product  Inputs=4
  p(t) : Outport
  wires:
  Constant/1 -> Product/1
  Constant1/1 -> Product/2
  Clock/1 -> Gain/1, Product/3
  Gain/1 -> Math Function/1
  Math Function/1 -> Product/4
  Product/1 -> Gain1/1
  Gain1/1 -> p(t)/1

== system regulator_de_stare/perturbatie38 ==
  Clock : Clock
  Constant : Constant  Value=Dg
  Constant1 : Constant  Value=Ag
  Gain : Gain  Gain=-1/tg_max
  Gain1 : Gain  Gain=1/(tg_max*tg_max)
  Math Function : Math
  Product : Product  Inputs=4
  p(t) : Outport
  wires:
  Constant/1 -> Product/1
  Constant1/1 -> Product/2
  Clock/1 -> Gain/1, Product/3
  Gain/1 -> Math Function/1
  Math Function/1 -> Product/4
  Product/1 -> Gain1/1
  Gain1/1 -> p(t)/1

== system regulator_de_stare/perturbatie39 ==
  Clock : Clock
  Constant : Constant  Value=Dg
  Constant1 : Constant  Value=Ag
  Gain : Gain  Gain=-1/tg_max
  Gain1 : Gain  Gain=1/(tg_max*tg_max)
  Math Function : Math
  Product : Product  Inputs=4
  p(t) : Outport
  wires:
  Constant/1 -> Product/1
  Constant1/1 -> Product/2
  Clock/1 -> Gain/1, Product/3
  Gain/1 -> Math Function/1
  Math Function/1 -> Product/4
  Product/1 -> Gain1/1
  Gain1/1 -> p(t)/1

== system regulator_de_stare/perturbatie4 ==
  Clock : Clock
  Constant : Constant  Value=Dg
  Constant1 : Constant  Value=Ag
  Gain : Gain  Gain=-1/tg_max
  Gain1 : Gain  Gain=1/(tg_max*tg_max)
  Math Function : Math
  Product : Product  Inputs=4
  p(t) : Outport
  wires:
  Constant/1 -> Product/1
  Constant1/1 -> Product/2
  Clock/1 -> Gain/1, Product/3
  Gain/1 -> Math Function/1
  Math Function/1 -> Product/4
  Product/1 -> Gain1/1
  Gain1/1 -> p(t)/1
